simulink model "HIL_Testing_SW"  (Simulink 7.5)
settings: Solver=ode1  StartTime=0.0  StopTime=Inf  FixedStep=0.001  RelTol=1e-3
PostLoadFcn:
  | , if any(exist('dsrtsu_mdlpostloadfcn', 'file') == [2, 3, 6]), try dsrtsu_mdlpostloadfcn('Execute', bdroot); catch fprintf('Error in PostLoadFcn (dsrtsu_mdlpostloadfcn) for model "%s":\n %s\n', bdroot, lasterr); end, end,
undefined symbols (not defined in the file): CeBSER_Cnt_NumTempAxisPts, ChargeCord, ChargeCord_Control, ChargeToSOCCurr, ChrgCurrLim, CrntSens1Fine, CS_SOCSetPt, CyclerMaxChrgPwr, CyclerMaxDschrgPwr, deltaAhr, Drive_1, Drive_10, Drive_11, Drive_12, Drive_13, Drive_14, Drive_15, Drive_16, Drive_17, Drive_18, Drive_19, Drive_2, Drive_20, Drive_21, Drive_22, Drive_23, Drive_24, Drive_25, Drive_26, Drive_27, Drive_28, Drive_29, Drive_3, Drive_30, Drive_31, Drive_32, Drive_33, Drive_34, Drive_35, Drive_36, Drive_37, Drive_38, Drive_39, Drive_4, Drive_40, Drive_41, Drive_42, Drive_43, Drive_44, Drive_45, Drive_46, Drive_47, Drive_48, Drive_49, Drive_5, Drive_50, Drive_51, Drive_6, Drive_7, Drive_8 ... (+50)
libraries: simulink x129, rtican x50, rti2211sailib x5, rti2211serlib x5, rti2202miolib x3
(part 21 of 23)

== system HIL_Testing_SW/LionsHeart/FeaturePresentation/Down_to_Business/DriveProfile_ModeControl/Drive_Profile/CD/Drive_49 ==
  loop_time : Inport  OutDataType=sfix(16)  OutScaling=2^0
  Enable : EnablePort
  Lookup Table : Lookup  InputValues=Drive_49(:,1)  Table=Drive_49(:,2)  OutDataType=fixdt(1, 16)  OutScaling=2^0
  Product1 : Product  OutDataType=sfix(16)  OutScaling=2^0  RndMeth=Zero
  W_kW : Constant  Value=single(1000)  OutDataType=sfix(16)  OutScaling=2^0
  Profile_Data : Outport  OutDataType=sfix(16)  OutScaling=2^0
  wires:
  loop_time/1 -> Lookup Table/1
  W_kW/1 -> Product1/2
  Lookup Table/1 -> Product1/1
  Product1/1 -> Profile_Data/1

== system HIL_Testing_SW/LionsHeart/FeaturePresentation/Down_to_Business/DriveProfile_ModeControl/Drive_Profile/CD/Drive_5 ==
  loop_time : Inport  OutDataType=sfix(16)  OutScaling=2^0
  Enable : EnablePort
  Lookup Table : Lookup  InputValues=Drive_5(:,1)  Table=Drive_5(:,2)  OutDataType=fixdt(1, 16)  OutScaling=2^0
  Product1 : Product  OutDataType=sfix(16)  OutScaling=2^0  RndMeth=Zero
  W_kW : Constant  Value=single(1000)  OutDataType=sfix(16)  OutScaling=2^0
  Profile_Data : Outport  OutDataType=sfix(16)  OutScaling=2^0
  wires:
  loop_time/1 -> Lookup Table/1
  W_kW/1 -> Product1/2
  Lookup Table/1 -> Product1/1
  Product1/1 -> Profile_Data/1

== system HIL_Testing_SW/LionsHeart/FeaturePresentation/Down_to_Business/DriveProfile_ModeControl/Drive_Profile/CD/Drive_50 ==
  loop_time : Inport  OutDataType=sfix(16)  OutScaling=2^0
  Enable : EnablePort
  Lookup Table : Lookup  InputValues=Drive_50(:,1)  Table=Drive_50(:,2)  OutDataType=fixdt(1, 16)  OutScaling=2^0
  Product1 : Product  OutDataType=sfix(16)  OutScaling=2^0  RndMeth=Zero
  W_kW : Constant  Value=single(1000)  OutDataType=sfix(16)  OutScaling=2^0
  Profile_Data : Outport  OutDataType=sfix(16)  OutScaling=2^0
  wires:
  Product1/1 -> Profile_Data/1
  Lookup Table/1 -> Product1/1
  W_kW/1 -> Product1/2
  loop_time/1 -> Lookup Table/1

== system HIL_Testing_SW/LionsHeart/FeaturePresentation/Down_to_Business/DriveProfile_ModeControl/Drive_Profile/CD/Drive_51 ==
  loop_time : Inport  OutDataType=sfix(16)  OutScaling=2^0
  Enable : EnablePort
  Lookup Table : Lookup  InputValues=Drive_51(:,1)  Table=Drive_51(:,2)  OutDataType=fixdt(1, 16)  OutScaling=2^0
  Product1 : Product  OutDataType=sfix(16)  OutScaling=2^0  RndMeth=Zero
  W_kW : Constant  Value=single(1000)  OutDataType=sfix(16)  OutScaling=2^0
  Profile_Data : Outport  OutDataType=sfix(16)  OutScaling=2^0
  wires:
  loop_time/1 -> Lookup Table/1
  W_kW/1 -> Product1/2
  Lookup Table/1 -> Product1/1
  Product1/1 -> Profile_Data/1

== system HIL_Testing_SW/LionsHeart/FeaturePresentation/Down_to_Business/DriveProfile_ModeControl/Drive_Profile/CD/Drive_6 ==
  loop_time : Inport  OutDataType=sfix(16)  OutScaling=2^0
  Enable : EnablePort
  Lookup Table : Lookup  InputValues=Drive_6(:,1)  Table=Drive_6(:,2)  OutDataType=fixdt(1, 16)  OutScaling=2^0
  Product1 : Product  OutDataType=sfix(16)  OutScaling=2^0  RndMeth=Zero
  W_kW : Constant  Value=single(1000)  OutDataType=sfix(16)  OutScaling=2^0
  Profile_Data : Outport  OutDataType=sfix(16)  OutScaling=2^0
  wires:
  Product1/1 -> Profile_Data/1
  Lookup Table/1 -> Product1/1
  W_kW/1 -> Product1/2
  loop_time/1 -> Lookup Table/1

== system HIL_Testing_SW/LionsHeart/FeaturePresentation/Down_to_Business/DriveProfile_ModeControl/Drive_Profile/CD/Drive_7 ==
  loop_time : Inport  OutDataType=sfix(16)  OutScaling=2^0
  Enable : EnablePort
  Lookup Table : Lookup  InputValues=Drive_7(:,1)  Table=Drive_7(:,2)  OutDataType=fixdt(1, 16)  OutScaling=2^0
  Product1 : Product  OutDataType=sfix(16)  OutScaling=2^0  RndMeth=Zero
  W_kW : Constant  Value=single(1000)  OutDataType=sfix(16)  OutScaling=2^0
  Profile_Data : Outport  OutDataType=sfix(16)  OutScaling=2^0
  wires:
  Product1/1 -> Profile_Data/1
  Lookup Table/1 -> Product1/1
  W_kW/1 -> Product1/2
  loop_time/1 -> Lookup Table/1

== system HIL_Testing_SW/LionsHeart/FeaturePresentation/Down_to_Business/DriveProfile_ModeControl/Drive_Profile/CD/Drive_8 ==
  loop_time : Inport  OutDataType=sfix(16)  OutScaling=2^0
  Enable : EnablePort
  Lookup Table : Lookup  InputValues=Drive_8(:,1)  Table=Drive_8(:,2)  OutDataType=fixdt(1, 16)  OutScaling=2^0
  Product1 : Product  OutDataType=sfix(16)  OutScaling=2^0  RndMeth=Zero
  W_kW : Constant  Value=single(1000)  OutDataType=sfix(16)  OutScaling=2^0
  Profile_Data : Outport  OutDataType=sfix(16)  OutScaling=2^0
  wires:
  Product1/1 -> Profile_Data/1
  Lookup Table/1 -> Product1/1
  W_kW/1 -> Product1/2
  loop_time/1 -> Lookup Table/1

== system HIL_Testing_SW/LionsHeart/FeaturePresentation/Down_to_Business/DriveProfile_ModeControl/Drive_Profile/CD/Drive_9 ==
  loop_time : Inport  OutDataType=sfix(16)  OutScaling=2^0
  Enable : EnablePort
  Lookup Table : Lookup  InputValues=Drive_9(:,1)  Table=Drive_9(:,2)  OutDataType=fixdt(1, 16)  OutScaling=2^0
  Product1 : Product  OutDataType=sfix(16)  OutScaling=2^0  RndMeth=Zero
  W_kW : Constant  Value=single(1000)  OutDataType=sfix(16)  OutScaling=2^0
  Profile_Data : Outport  OutDataType=sfix(16)  OutScaling=2^0
  wires:
  loop_time/1 -> Lookup Table/1
  W_kW/1 -> Product1/2
  Lookup Table/1 -> Product1/1
  Product1/1 -> Profile_Data/1

== system HIL_Testing_SW/LionsHeart/FeaturePresentation/Down_to_Business/DriveProfile_ModeControl/Drive_Profile/CD/Magic ==
  note: upper
  note: Lower
  InputPower : Inport  OutDataType=fixdt(1, 16)  OutScaling=2^0
  EndTime : Inport  Port=2  OutDataType=fixdt(1, 16)  OutScaling=2^0
  LoopTime : Inport  Port=3  OutDataType=fixdt(1, 16)  OutScaling=2^0
  CD_Lo : Constant  Value=-80  OutDataType=fixdt(1, 16)  OutScaling=2^0
  CD_Up : Constant  Value=.5  OutDataType=fixdt(1, 16)  OutScaling=2^0
  CI_Lo : Constant  Value=-.5  OutDataType=fixdt(1, 16)  OutScaling=2^0
  CI_Up : Constant  Value=10  OutDataType=fixdt(1, 16)  OutScaling=2^0
  CS_Lo : Constant  Value=-5  OutDataType=fixdt(1, 16)  OutScaling=2^0
  CS_Up : Constant  Value=5  OutDataType=fixdt(1, 16)  OutScaling=2^0
  Compare To Zero : simulink/Logic and Bit Operations/Compare To Zero  SystemSampleTime=-1  relop=>=  LogicOutDataTypeMode=uint8
  Compare To Zero1 : simulink/Logic and Bit Operations/Compare To Zero  SystemSampleTime=-1  relop=>  LogicOutDataTypeMode=uint8
  Compare To Zero2 : simulink/Logic and Bit Operations/Compare To Zero  SystemSampleTime=-1  relop=>=  LogicOutDataTypeMode=uint8
  Compare To Zero3 : simulink/Logic and Bit Operations/Compare To Zero  SystemSampleTime=-1  relop=<  LogicOutDataTypeMode=uint8
  Constant{,1..2,4} (4 alike) : Constant  OutDataType=fixdt(1, 16)  OutScaling=2^0
  Constant3 : Constant  Value=.001  OutDataType=fixdt(1, 16)  OutScaling=2^0
  Data Store Read : DataStoreRead  DataStoreName=ProfileDynamicGainEnable  SampleTime=0
  Data Store Read1 : DataStoreRead  DataStoreName=ProfileChargeDesignation  SampleTime=0
  Data Store Read2 : DataStoreRead  DataStoreName=ProfileChargeDesignation  SampleTime=0
  Data Store Read3 : DataStoreRead  DataStoreName=Ahr  SampleTime=0
  Divide : Product  Inputs=*/  OutDataType=fixdt(1, 16)  OutScaling=2^-10
  Divide1 : Product  Inputs=*/  OutDataType=fixdt(1, 16)  OutScaling=2^-10
  Lookup Table1 : Lookup  InputValues=[.1 .5 .75 1 2]  Table=[-.5 0 .5 1 1]  OutDataType=fixdt(1, 16)  OutScaling=2^0
  Lookup Table2 : Lookup  InputValues=[.1 .5 .75 1 2]  Table=[-.5 0 .5 1 1]  OutDataType=fixdt(1, 16)  OutScaling=2^0
  Multiport Switch : MultiPortSwitch  zeroidx=off  OutDataType=fixdt(1, 16)  OutScaling=2^0
  Multiport Switch1 : MultiPortSwitch  zeroidx=off  OutDataType=fixdt(1, 16)  OutScaling=2^0
  Product : Product  OutDataType=fixdt(1, 16)  OutScaling=2^0  RndMeth=Zero
  Product1 : Product  OutDataType=fixdt(1, 16)  OutScaling=2^0  OutDataTypeStr=Inherit: Inherit via back propagation  RndMeth=Zero
  Relational Operator : RelationalOperator  Operator===  LogicOutDataTypeMode=boolean  LogicDataType=fixdt(0, 8)  OutDataTypeStr=boolean
  Saturation : Saturate  UpperLimit=1  LowerLimit=-1  OutDataType=fixdt(1, 16)  OutScaling=2^0
  Saturation1 : Saturate  UpperLimit=1  LowerLimit=-1  OutDataType=fixdt(1, 16)  OutScaling=2^0
  Subtract : Sum  Inputs=+-+  OutDataType=fixdt(1, 16)  OutScaling=2^-10
  Switch{,1..2,4..5} (5 alike) : Switch  Threshold=.5  OutDataType=fixdt(1, 16)  OutScaling=2^0
  Switch3 : Switch  Threshold=.5  OutDataType=fixdt(1, 16)  OutScaling=2^0  OutDataTypeStr=Inherit: Inherit via back propagation
  Unit Delay : UnitDelay  SampleTime=-1
  ProfileData : Outport  OutDataType=fixdt(1, 16)  OutScaling=2^0
  wires:
  InputPower/1 -> [InPower]
  EndTime/1 -> Relational Operator/1
  LoopTime/1 -> Relational Operator/2
  Relational Operator/1 -> Switch/2
  [Ahr] -> Switch/1
  Switch/1 -> [AhrOld], Unit Delay/1
  Unit Delay/1 -> Switch/3
  [Ahr] -> Subtract/1
  [AhrOld] -> Subtract/2
  Subtract/1 -> [AhrInternal]
  [InPower] -> Compare To Zero/1
  Compare To Zero/1 -> Switch1/2
  Constant/1 -> Switch1/1
  Constant1/1 -> Switch1/3
  [InPower] -> Product/2
  [InPower] -> Compare To Zero2/1
  Compare To Zero2/1 -> Switch2/2
  [ChargeGain] -> Switch2/1
  Switch1/1 -> Product/1
  CI_Up/1 -> Multiport Switch/2
  CS_Up/1 -> Multiport Switch/3
  CD_Up/1 -> Multiport Switch/4
  Data Store Read1/1 -> Multiport Switch/1
  Data Store Read2/1 -> Multiport Switch1/1
  CI_Lo/1 -> Multiport Switch1/2
  CS_Lo/1 -> Multiport Switch1/3
  CD_Lo/1 -> Multiport Switch1/4
  Multiport Switch/1 -> Divide/1
  Saturation/1 -> [ChargeGain]
  Multiport Switch1/1 -> Divide1/1
  Saturation1/1 -> [DisChargeGain]
  [DisChargeGain] -> Switch2/3
  Product/1 -> Switch3/1, [PowerTemp]
  [PowerTemp] -> Product1/2
  Switch2/1 -> Product1/1
  Product1/1 -> Switch3/3
  Switch3/1 -> ProfileData/1
  Constant3/1 -> Subtract/3
  Data Store Read/1 -> Switch3/2
  Data Store Read3/1 -> [Ahr]
  [AhrInternal] -> Compare To Zero1/1
  Compare To Zero1/1 -> Switch4/2
  Constant2/1 -> Switch4/3
  [AhrInternal] -> Compare To Zero3/1
  Compare To Zero3/1 -> Switch5/2
  Constant4/1 -> Switch5/3
  [AhrInternal] -> Divide/2
  Divide/1 -> Switch4/1
  Switch4/1 -> Lookup Table2/1
  Lookup Table2/1 -> Saturation/1
  [AhrInternal] -> Divide1/2
  Divide1/1 -> Switch5/1
  Switch5/1 -> Lookup Table1/1
  Lookup Table1/1 -> Saturation1/1

== stateflow chart RX/Read BAS3/PID_Reads/Chart ==
  state Zach
    en: Increment = Increment +1;
  state Initialize
    en:Increment =1;
  state Zac
    en: Increment = Increment +1;
  (default) -> Initialize
  Initialize -> Zach : after(Timer,sec)
  Zach -> Zac : after(Timer,sec)
  Zac -> Initialize : after(Timer,sec)
  data: Timer input double; Increment output double

== stateflow chart TX/Tx_Cycler/TX_ABC_ChA/Chart ==
  state Zach
    en:Trigger_one =1;
    ex:Trigger_one = 0;
  state Zachashley
    en:Trigger_two = 1;
    ex:Trigger_two = 0;
  state ashley
    en:Trigger_three = 1;
    ex:Trigger_three = 0;
    Increment = Increment +1;
  state Reset
    en:Increment =1;
  state Initialize
    en:Increment =1;
  state Zach2
  state Zachashley2
  state ashley2
  (default) -> Initialize
  Zach2 -> Zachashley : after(TickTick,tick)
  Zachashley2 -> ashley : after(TickTick,tick)
  ashley2 -> Zach : after(TickTick,tick)
  ashley -> Reset [order 1] : [Increment >254]
  Initialize -> Zach
  Reset -> Zach
  Zach -> Zach2
  Zachashley -> Zachashley2
  ashley -> ashley2 [order 2]
  data: Trigger_one output double; Trigger_two output double; Trigger_three output double; TickTick input double; Increment output double

== stateflow chart TX/Tx_Cycler/TX_ABC_ChB/Chart ==
  state Zach
    en:Trigger_one =1;
    ex:Trigger_one = 0;
  state Zachashley
    en:Trigger_two = 1;
    ex:Trigger_two = 0;
  state ashley
    en:Trigger_three = 1;
    ex:Trigger_three = 0;
    Increment = Increment +1;
  state Reset
    en:Increment =1;
  state Initialize
    en:Increment =1;
  state Zach2
  state Zachashley2
  state ashley2
  (default) -> Initialize
  Zach2 -> Zachashley : after(TickTick,tick)
  Zachashley2 -> ashley : after(TickTick,tick)
  ashley2 -> Zach : after(TickTick,tick)
  ashley -> Reset [order 1] : [Increment >254]
  Initialize -> Zach
  Reset -> Zach
  Zach -> Zach2
  Zachashley -> Zachashley2
  ashley -> ashley2 [order 2]
  data: Trigger_one output double; Trigger_two output double; Trigger_three output double; TickTick input double; Increment output double

== stateflow chart TX/Tx_Cycler/Take_Cycler_Command ==
  state Handshake
    state Handshake_Done
      en: Handshake_Complete=1;
    state Hold2
    state Ping
      en: Send_Ping=1;
      exit: Send_Ping=0;
    state Hold1
    state Greeting
      en: Send_Greeting=1;
      exit: Send_Greeting=0;
    Handshake_Done -> Handshake
    (default) -> Ping
    Hold1 -> Greeting : after(500,tick)
    Ping -> Hold1 : [(Version~=0)&&(Hardware~=0)]
    Hold2 -> Handshake_Done : after(500,tick)
    Greeting -> Hold2 : [Greeting_Sent==1]
  state Init
    en:
    Send_Ping=0;
    Send_Greeting=0;
    Send_Remote_Req_B=0;
    Send_Commands=0;
    Greeting_Sent=0;
    Remote_Req_B_Sent=0;
  state Finish
    en:
    Send_Commands=1;
  state Remote
    en:
    Channel_Change_B=Channel;
    Control_From_B=0;
    Control_To_B=1;
    Send_Remote_Req_B=1;
    exit: Send_Remote_Req_B=0;
  state Local
    en:
    Handshake_Complete = 0;
    Channel_Change_B=Channel;
    Control_From_B=1;
    Control_To_B=0;
    Send_Remote_Req_B=1;
    exit: Send_Remote_Req_B=0;
  state Wait
    en:
    Send_Ping=0;
    Send_Greeting=0;
    Send_Remote_Req_B=0;
    Send_Commands=0;
    Greeting_Sent=0;
    Remote_Req_B_Sent=0;
    Handshake_Complete = 0;
  Remote -> Handshake [order 1] : after(5000,tick)[(Remote_Req_B_Sent)&&(Side_B_Status==0)]
  Remote -> Finish [order 2] : after(100,tick)[(Remote_Req_B_Sent==1)&&(Side_B_Status==1)]
  Handshake -> Remote : [(Handshake_Complete==1)&&(Status==1)]
  (default) -> Init
  Init -> Handshake : [Perform_Handshake]
  Finish -> Local : [Reset_to_Local == 1]
  Local -> Wait : [Side_B_Status==0]
  Wait -> Handshake : [Perform_Handshake]
  data: Version input double; Hardware input double; Status input double; Send_Ping output double; Send_Greeting output double; Greeting_Sent data_store_memory double; Send_Remote_Req_B output double; Side_B_Status input double; Perform_Handshake input boolean; Handshake_Complete data_store_memory double; Remote_Req_B_Sent data_store_memory double; Channel_Change_B output double; Control_From_B output double; Control_To_B output double; Send_Commands output double =0; Reset_to_Local input boolean; Channel input double

== stateflow chart TX/Chiller/ChillerCmndTxDecision/ChillerStateFlow ==
  state EvaluateChillerOnOff
  state ManualSelect
    en:
    WaitRx = 1;
    ChillerTx = ManualChillerSP_Cmnd;
    ChillerTxNumBytes = 8;
    ChillerRxNumBytes = 2;
    exit:
    ChillerTxNumBytes = 0;
  state ReadChillerSP2
    en:
    exit:
    ReadChillerSP_Action = 0;
  state TurnChillerOff
    en:
    WaitRx = 1;
    ChillerTx = TurnChiller_Off;
    ChillerTxNumBytes = 4;
    ChillerRxNumBytes = 2;
  state GoBack
  state ReadChillerTemp2
    en:
    exit:
    ReadChillerTemp_Action = 0;
  state ManualSelect1
    en:
    exit:
    ChillerTxNumBytes = 0;
    WaitRx = 0;
  state ReadChillerStatus1
    en:
    WaitRx = 0;
    ReadChillerStatus_Action = 1;
    ChillerTx = ReadChillerStatus;
    ChillerTxNumBytes = 3;
    ChillerRxNumBytes = 2;
  state ReadChillerSP1
    en:
    ChillerTx = ReadChillerSP;
    ChillerTxNumBytes = 3;
    ChillerRxNumBytes = 7;
    ReadChillerSP_Action = 1;
    exit:
    ChillerTxNumBytes = 0;
  state ReadChillerTemp1
    en:
    ReadChillerTemp_Action = 1;
    ChillerTx = ReadChillerTemp;
    ChillerTxNumBytes = 3;
    ChillerRxNumBytes = 7;
    exit:
    ChillerTxNumBytes = 0;
  state EvaluateBatTemp3
    en:
    WaitRx = 1;
    ChillerTx = TurnChiller_On;
    ChillerTxNumBytes = 4;
    ChillerRxNumBytes = 2;
    exit:
    ChillerTxNumBytes = 0;
  state EvaluateBatTemp4
    en:
    WaitRx = 0;
    ChillerTxNumBytes = 0;
    ChillerRxNumBytes = 0;
    ChillerPowerStatus = 0;
  state ReadChillerStatus
    en:
    exit:
    ReadChillerStatus_Action = 0;
    ChillerPowerStatus = 1;
  state FollowProfileTemp
    en:
    WaitRx = 1;
    ChillerTx =  BatTempSwitchSlct;
    ChillerTxNumBytes = 8;
    ChillerRxNumBytes = 2;
    exit:
    ChillerTxNumBytes = 0;
  (default) -> EvaluateBatTemp4
  EvaluateBatTemp4 -> EvaluateBatTemp3 [order 1] : [(ChillerOnOff == 1 && (BatTemp > 33 || BatTemp < 0) && ChillerOpMode ==1)]
  EvaluateChillerOnOff -> FollowProfileTemp [order 2] : [(ChillerOpMode == 1 && (BatTemp > 33 || BatTemp < 0))]
  EvaluateChillerOnOff -> ManualSelect [order 4] : [ChillerOpMode == 3&&ManualChillerPower ==1]
  EvaluateChillerOnOff -> ManualSelect [order 3] : [(ChillerOpMode == 2&&ManualChillerPower ==1)]
  ManualSelect1 -> ReadChillerSP1
  EvaluateChillerOnOff -> TurnChillerOff [order 1] : [(ChillerOnOff == 0)&&(ChillerOpMode == 1)]
  ReadChillerTemp1 -> ReadChillerTemp2
  ReadChillerSP2 -> ReadChillerTemp1
  ManualSelect -> ManualSelect1 : [PositiveResponse == 1]
  EvaluateBatTemp3 -> ReadChillerStatus1 : [PositiveResponse == 1]
  TurnChillerOff -> EvaluateBatTemp4 : [PositiveResponse == 1]
  ReadChillerSP1 -> ReadChillerSP2
  (junction 123) -> EvaluateChillerOnOff
  GoBack -> EvaluateChillerOnOff
  EvaluateChillerOnOff -> TurnChillerOff [order 6] : [(ChillerOpMode == 1 && BatTemp >= 0 && BatTemp < 33)]
  FollowProfileTemp -> ManualSelect1 : [PositiveResponse == 1]
  ReadChillerStatus1 -> ReadChillerStatus : [ChillerOn == 1]
  ReadChillerStatus -> (junction 122)
  (junction 122) -> (junction 123)
  EvaluateBatTemp4 -> EvaluateBatTemp3 [order 2] : [ChillerOpMode == 3]
  ReadChillerTemp2 -> GoBack
  EvaluateChillerOnOff -> TurnChillerOff [order 5] : [ManualChillerPower == 0]
  EvaluateBatTemp4 -> EvaluateBatTemp3 [order 3] : [ManualChillerPower == 1]
  data: BatTempSwitchSlct input uint8 size=8; ManualChillerSP_Cmnd input uint8 size=8; ChillerTx output uint8 size=8; ChillerTxNumBytes output uint32; ChillerRxNumBytes output uint32; ReadChillerSP_Action output boolean; ChillerOnOff input boolean; ChillerOpMode input uint8; TurnChiller_On input uint8 size=8; TurnChiller_Off input uint8 size=8; ReadChillerSP input uint8 size=8; ReadChillerTemp input uint8 size=8; ReadChillerTemp_Action output boolean; PositiveResponse input boolean size=1; ReadChillerStatus input uint8 size=8; ChillerOn input boolean; ReadChillerStatus_Action output boolean; ManualChillerPower input boolean; ChillerPowerStatus output boolean; WaitRx output boolean; BatTemp input single

== stateflow chart LionsHeart/FeaturePresentation/Down_to_Business/DriveProfile_ModeControl/Capacity Test/Capacity_Test ==
  state ChargeTerminate
    entry:
    Mode_Cntrl_cap = 1;
    Step=5;
    WaitTime=0;
    RateInternal = RateInternal*RateFactor;
    ChrgCurrLim_Tmp=RateInternal;
    Control_Value_cap = RateInternal;
    du:
    WaitTime=WaitTime+sim_step_time;
    ChrgCurrLim_Tmp=RateInternal;
    Control_Value_cap = RateInternal;
    Cappy = 7;
  state DischargeTerminate
    entry:
    WaitTime = 0;
    Mode_Cntrl_cap = 1;
    Step=2;
    RateInternal = RateInternal*RateFactor;
    DischrgCurrLim_Tmp = RateInternal;
    Control_Value_cap = RateInternal
    du:
    DischrgCurrLim_Tmp = RateInternal;
    Control_Value_cap = RateInternal;
    WaitTime=WaitTime+sim_step_time;
    Cappy = 3;
  state Taper
    entry:
    WaitTime = 0;
    du:
    WaitTime = WaitTime + sim_step_time;
    Cappy = 4;
  state Rest2
    entry:
    ResetSOCFlg = 1;
    Mode_Cntrl_cap = 3;
    WaitTime =0;
    Step=6;
    during:
    ResetSOCFlg = 0;
    WaitTime = WaitTime + sim_step_time;
    Cappy = 9;
    exit:
    cycle = cycle+1;
  state end_test
    entry:
    Step=99;
    Mode_Cntrl_cap = 3;
    DischrgCurrLim_Tmp=DischrgCurrLim;
    ChrgCurrLim_Tmp=ChrgCurrLim;
  state Taper_Charge
    entry:
    WaitTime = 0;
    du:
    WaitTime = WaitTime + sim_step_time;
    Cappy = 8;
  state Charge
    entry:
    Mode_Cntrl_cap = 1;
    Step=4;
    WaitTime=0;
    du:
    RateInternal = CRate;
    WaitTime=WaitTime+sim_step_time;
    ChrgCurrLim_Tmp=CRate;
    Control_Value_cap = CRate;
    Cappy = 6;
  state start_test
    entry:
    Step=0;
    cycle = 0;
    Mode_Cntrl_cap = 3;
    WaitTime = 0;
    DischrgCurrLim_Tmp=DischrgCurrLim;
    ChrgCurrLim_Tmp=ChrgCurrLim;
    ContactorOverride =1;
    du:
    WaitTime=WaitTime+sim_step_time;
    Cappy = 1;
  state Rest
    entry:
    ResetSOCFlg = 1;
    Mode_Cntrl_cap = 3;
    WaitTime =0;
    Step=3;
    during:
    WaitTime = WaitTime + sim_step_time;
    Cappy = 5;
    ResetSOCFlg = 0;
  state discharge
    entry:
    WaitTime = 0;
    Mode_Cntrl_cap = 1;
    Step=1;
    DischrgCurrLim_Tmp = -1*CRate;
    Control_Value_cap = -1*CRate;
    du:
    RateInternal = -1*CRate;
    DischrgCurrLim_Tmp = -1*CRate;
    Control_Value_cap = -1*CRate;
    WaitTime=WaitTime+sim_step_time;
    Cappy = 2;
  (default) -> start_test
  ChargeTerminate -> Rest2 [order 1] : [((Current_Cntrl<=CurrentTerm) && (WaitTime >=2)) || (CyclerVoltage > Vlid)]
  Taper_Charge -> ChargeTerminate [order 2] : [((Voltage_Cntrl>=Vlid) || ((PackVolt_MaxCell>=Vlid_cell) && (MaxCell_Enbl == 1))) && WaitTime > .5]
  ChargeTerminate -> Taper_Charge [order 2]
  DischargeTerminate -> Rest [order 1] : [((Current_Cntrl >=-1*CurrentTerm) && (WaitTime >= .5)) || (CyclerVoltage< Vfloor)]
  DischargeTerminate -> Taper [order 2]
  Taper -> DischargeTerminate [order 2] : [((Voltage_Cntrl<=Vfloor) || ((PackVolt_MinCell <=Vfloor_cell) && MinCell_Enbl == 1)) && (WaitTime > .5)]
  Rest2 -> discharge [order 2] : [ (WaitTime >= RestTime) && (cycle<NumberCycles)]
  discharge -> Rest [order 2] : [((Voltage_Cntrl<= Vfloor) || ((PackVolt_MinCell <=Vfloor_cell) && (MinCell_Enbl == 1))) && (Vfloor != OCV_Zero)]
  Rest -> Charge : [ WaitTime >= RestTime]
  discharge -> DischargeTerminate [order 1] : [((Voltage_Cntrl<=Vfloor) || ((PackVolt_MinCell <=Vfloor_cell) && (MinCell_Enbl == 1))) && (Vfloor == OCV_Zero)]
  start_test -> discharge : [ (cycle < NumberCycles) && (WaitTime>=30)]
  Charge -> ChargeTerminate : [(Voltage_Cntrl>=Vlid) || ((PackVolt_MaxCell>=Vlid_cell) && (MaxCell_Enbl == 1))]
  Rest2 -> end_test [order 1] : [(WaitTime >= RestTime) && (cycle>=NumberCycles)]
  Taper -> Rest [order 1] : [Current_Cntrl >=-1*CurrentTerm]
  Taper_Charge -> Rest2 [order 1] : [Current_Cntrl<=CurrentTerm]
  data: Control_Value_cap output double; Vfloor input single; WaitTime output double; Mode_Cntrl_cap output single; Vlid input single; CurrentTerm input single; Voltage_Cntrl input single; Current_Cntrl input single; NumberCycles input single; sim_step_time input single; cycle output single; RestTime input single; ChrgCurrLim input single; DischrgCurrLim input single; DischrgCurrLim_Tmp output single; ChrgCurrLim_Tmp output single; Step output single; PackVolt_MinCell input double; PackVolt_MaxCell input double; RateFactor input single; Vfloor_cell input double; Vlid_cell input double; MaxCell_Enbl input double; MinCell_Enbl input double; CyclerVoltage input double; RateInternal local double; OCV_Zero input double; CRate input double; ContactorOverride output double; Cappy output int32; ResetSOCFlg output boolean

== stateflow chart LionsHeart/FeaturePresentation/Down_to_Business/DriveProfile_ModeControl/Charging_Mode/Charging Logic1 ==
  state WaitBlock2
    Step =7;
    WaitTime = 0;
    du:
    WaitTime = WaitTime + sim_step_time;
  state CheckDirectionVoltage
    entry:
    Mode_Cntrl_cap=3;
  state Pack_Sens_Termination3
    entry:
    Mode_Cntrl_cap = 3;
    WaitTime= 0;
    Step=0;
    du:
    WaitTime=WaitTime+sim_step_time;
    DisChrgCurr_Limit = DisChrgCurrLimit_Cal;
    ChargeLimit_Temp = ChargeLimitCal;
  state Pack_Sens_DschrgTerminate
    entry:
    Mode_Cntrl_cap = 1;
    Step=6;
    RateDschrg= RateDschrg*RateFactor;
    Control_Value_cap = RateDschrg;
    du:
    Control_Value_cap = RateDschrg;
  state Pack_Sens_Discharge
    entry:
    RateChrgInternal = RateChrg;
    RateDschrg = RateChrg*-1;
    DisChrgCurr_Limit = RateDschrg;
    ChargeLimit_Temp = RateChrgInternal;
    Mode_Cntrl_cap = 1;
    Step=2;
    du:
    Control_Value_cap = RateDschrg;
  state Decision_Block
    Mode_Cntrl_cap = 3;
  state Pack_Sens_Termination2
    entry:
    Step=99;
    Mode_Cntrl_cap = 3;
    DisChrgCurr_Limit = DisChrgCurrLimit_Cal;
    ChargeLimit_Temp = ChargeLimitCal;
    du:
    Mode_Cntrl_cap = 3;
    DisChrgCurr_Limit = DisChrgCurrLimit_Cal;
    ChargeLimit_Temp = ChargeLimitCal;
  state Pack_Sens_Termination
    entry:
    Mode_Cntrl_cap = 1;
    Step=6;
    RateChrgInternal = RateChrgInternal *RateFactor;
    Control_Value_cap = RateChrgInternal;
    du:
    Control_Value_cap = RateChrgInternal;
  state Pack_Sens_Termination1
    entry:
    RateChrgInternal = RateChrg;
    DisChrgCurr_Limit = RateChrgInternal*-1;
    ChargeLimit_Temp = RateChrgInternal;
    Mode_Cntrl_cap = 1;
    Step=2;
    du:
    RateChrgInternal = RateChrg;
    Control_Value_cap = RateChrgInternal;
  state WaitBlock1
    Step =7;
    WaitTime = 0;
    du:
    WaitTime = WaitTime + sim_step_time;
  state CheckDirectionSOC
    entry:
    Mode_Cntrl_cap=3;
  state Termination_SOC
    entry:
    Step=99;
    Mode_Cntrl_cap = 3;
    DisChrgCurr_Limit = DisChrgCurrLimit_Cal;
    ChargeLimit_Temp = ChargeLimitCal;
    du:
    Mode_Cntrl_cap = 3;
    DisChrgCurr_Limit = DisChrgCurrLimit_Cal;
    ChargeLimit_Temp = ChargeLimitCal;
  state TaperToCurrentTerm_SOC
    entry:
    Mode_Cntrl_cap = 1;
    Step=6;
    RateChrgInternal = RateChrgInternal *RateFactor;
    Control_Value_cap = RateChrgInternal;
    du:
    Control_Value_cap = RateChrgInternal;
  state ChargeToSOC
    entry:
    RateChrgInternal = RateChrg;
    DisChrgCurr_Limit = RateChrgInternal*-1;
    ChargeLimit_Temp = RateChrgInternal;
    Mode_Cntrl_cap = 1;
    Step=2;
    du:
    RateChrgInternal = RateChrg;
    Control_Value_cap = RateChrgInternal;
  state WaitBlock3
    Step =7;
    WaitTime = 0;
    du:
    WaitTime = WaitTime + sim_step_time;
  state WaitBlock4
    Step =7;
    WaitTime = 0;
    du:
    WaitTime = WaitTime + sim_step_time;
  state Pack_Sens_DschrgTerminate1
    entry:
    Mode_Cntrl_cap = 1;
    Step=6;
    RateDschrg= RateDschrg*RateFactor;
    Control_Value_cap = RateDschrg;
    du:
    Control_Value_cap = RateDschrg;
  state DischargeToSOC
    entry:
    RateChrgInternal = RateChrg;
    RateDschrg = RateChrg*-1;
    DisChrgCurr_Limit = RateDschrg;
    ChargeLimit_Temp = RateChrgInternal;
    Mode_Cntrl_cap = 1;
    Step=2;
    du:
    Control_Value_cap = RateDschrg;
  (default) -> Decision_Block
  Pack_Sens_DschrgTerminate -> Pack_Sens_Termination2 [order 1] : [(Current_Cntrl>=-1*CurrentTerm) || (CyclerVoltage<VFloor)]
  Pack_Sens_Termination3 -> CheckDirectionVoltage [order 2] : [(WaitTime >= WaitTime1) && ((ChargeSelect == 0) || (ChargeSelect==1))]
  Pack_Sens_DschrgTerminate -> WaitBlock2 [order 2]
  CheckDirectionVoltage -> Pack_Sens_Termination1 [order 1] : [Voltage_Cntrl<=VoltageSetPoint]
  WaitBlock2 -> Pack_Sens_DschrgTerminate [order 2] : [((PackVoltage_MinCell<=VoltageSetPoint) && (MinCell_Enbl == 1)) || (CyclerVoltage <= VoltageSetPoint) || (Voltage_Cntrl<=VoltageSetPoint)&& (WaitTime > .5)]
  Pack_Sens_Discharge -> Pack_Sens_DschrgTerminate : [((PackVoltage_MinCell<=VoltageSetPoint) && (MinCell_Enbl == 1)) || (CyclerVoltage <= VoltageSetPoint) || (Voltage_Cntrl<=VoltageSetPoint)]
  CheckDirectionVoltage -> Pack_Sens_Discharge [order 2] : [Voltage_Cntrl>VoltageSetPoint]
  WaitBlock1 -> Pack_Sens_Termination [order 2] : [(((PackVoltage_MaxCell>=VoltageSetPt_Max) && (MaxCell_Enbl == 1)) || (CyclerVoltage>=(VoltageSetPoint+CyclerOffset)) || (Voltage_Cntrl >= VoltageSetPoint)) && (WaitTime > .5)]
  Pack_Sens_Termination -> Pack_Sens_Termination2 [order 1] : [(Current_Cntrl<CurrentTerm) || (CyclerVoltage>(VoltageLid+CyclerOffset))]
  Pack_Sens_Termination1 -> Pack_Sens_Termination : [((PackVoltage_MaxCell >= VoltageSetPt_Max) && (MaxCell_Enbl ==1)) || (CyclerVoltage >= VoltageSetPoint) || (Voltage_Cntrl >=VoltageSetPoint)]
  Pack_Sens_Termination -> WaitBlock1 [order 2]
  Decision_Block -> Pack_Sens_Termination3
  WaitBlock1 -> Pack_Sens_Termination2 [order 1] : [Current_Cntrl<CurrentTerm]
  WaitBlock2 -> Pack_Sens_Termination2 [order 1] : [Current_Cntrl>=-1*CurrentTerm]
  Pack_Sens_Termination3 -> CheckDirectionSOC [order 1] : [(WaitTime >= WaitTime1) && (ChargeSelect == 2)]
  CheckDirectionSOC -> ChargeToSOC [order 1] : [SOC<=SOCTarget]
  WaitBlock3 -> TaperToCurrentTerm_SOC [order 2] : [((SOC>=SOCTarget) && (WaitTime > .5))]
  TaperToCurrentTerm_SOC -> Termination_SOC [order 1] : [(Current_Cntrl<CurrentTerm) || (CyclerVoltage>VoltageLid)]
  ChargeToSOC -> TaperToCurrentTerm_SOC : [SOC>=SOCTarget]
  TaperToCurrentTerm_SOC -> WaitBlock3 [order 2]
  WaitBlock3 -> Termination_SOC [order 1] : [Current_Cntrl<CurrentTerm]
  CheckDirectionSOC -> Termination_SOC [order 2] : [SOC >! 0]
  Pack_Sens_DschrgTerminate1 -> Termination_SOC [order 1] : [(Current_Cntrl>=-1*CurrentTerm) || (CyclerVoltage<VFloor)]
  Pack_Sens_DschrgTerminate1 -> WaitBlock4 [order 2]
  WaitBlock4 -> Pack_Sens_DschrgTerminate1 [order 2] : [((SOC<=SOCTarget) && (WaitTime > .5))]
  DischargeToSOC -> Pack_Sens_DschrgTerminate1 : [SOC<=SOCTarget]
  CheckDirectionSOC -> DischargeToSOC [order 3] : [SOC>SOCTarget]
  WaitBlock4 -> Termination_SOC [order 1] : [Current_Cntrl>=-1*CurrentTerm]
  data: Control_Value_cap output double; WaitTime output double; RateChrg input single; Mode_Cntrl_cap output single; VoltageSetPoint input single; CurrentTerm input single; Current_Cntrl input single; sim_step_time input single; WaitTime1 input single; ChargeSelect input single; SOC input double; VoltageLid input single; ChargeLimitCal input single; ChargeLimit_Temp output single; DisChrgCurr_Limit output single; DisChrgCurrLimit_Cal input single; Step output double; RateChrgInternal local double; CyclerVoltage input single; SOCTarget input double; RateFactor input single; VFloor input single; PackVoltage_MaxCell input double; PackVoltage_MinCell input double; RateDschrg local double; VoltageSetPt_Max input double; Voltage_Cntrl input double; MaxCell_Enbl input double; MinCell_Enbl input double; CyclerOffset input double

== stateflow chart LionsHeart/FeaturePresentation/Down_to_Business/DriveProfile_ModeControl/Drive_Profile/CD/Power_Cycle_Timer ==
  state start_dvr
    entry:
    loop_counter = 0;
    loop_time = 0;
  state run_cycle
    entry:loop_time = StartTime;
    during:
    loop_time = loop_time + sim_time_step;
    exit:
    loop_time = 0;
  state End_Test
    entry:
    loop_time = 0;
  state run_cycle1
    during:
    loop_time = loop_time + sim_time_step;
    exit:
    loop_time = 0;
  (default) -> start_dvr
  run_cycle -> start_dvr [order 1] : [ cycle_enable == 0]
  run_cycle -> End_Test [order 2] : [ loop_time >= cycle_duration ]
  start_dvr -> run_cycle [order 1] : [ (cycle_enable  == 1) && (StartTime~=0) ]
  End_Test -> start_dvr : [ cycle_enable == 0]
  start_dvr -> run_cycle1 [order 2] : [(cycle_enable==1) && (StartTime==0)]
  run_cycle1 -> start_dvr [order 1] : [cycle_enable ==0]
  run_cycle1 -> End_Test [order 2] : [loop_time>=cycle_duration]
  data: loop_counter output double; cycle_enable input boolean; sim_time_step input double; cycle_duration input double; loop_time output double; StartTime input double

== stateflow chart LionsHeart/FeaturePresentation/Down_to_Business/DriveProfile_ModeControl/HPPC Test/HPPC_Test ==
  state start_test
    entry:
    cycle = 0;
    ChrgCurrLim_Tmp=ChrgCurrLim;
  state Rest
    entry:
    RestTime =0;
    Mode_Cntrl = 3;
    Step=2;
    during:
    RestTime = RestTime + sim_step_time;
  state First_Discharge
    entry:
    EndTime = 0;
    during:
    Mode_Cntrl = 1;
    Step=3;
    Control_Value = RateDischrg;
    EndTime = EndTime + sim_step_time;
  state Discharge_Pulse
    entry:
    PulseTime=0;
    Step=4;
    du:
    Mode_Cntrl = 1;
    Control_Value = DischrgPulseCurr;
    PulseTime = PulseTime + sim_step_time;
  state Charge_Pulse
    entry:
    PulseTime =0;
    Step=4;
    during:
    PulseTime = PulseTime + sim_step_time;
    Mode_Cntrl = 1;
    Control_Value = ChrgPulseCurr;
  state Rest_Btwn_Pulse
    entry:
    RestBtwnTime =0;
    Mode_Cntrl = 3;
    Step=2;
    during:
    RestBtwnTime = RestBtwnTime + sim_step_time;
  state end_test
    entry:
    Mode_Cntrl = 3;
    Step=7;
  state Rest_Before
    entry:
    RestBefore =0;
    Mode_Cntrl = 3;
    Step=2;
    during:
    RestBefore = RestBefore + sim_step_time;
  state Discharge%
    entry:
    EndTime2 = 0;
    Step=3;
    during:
    Mode_Cntrl = 1;
    Control_Value = RateDischrg;
    EndTime2 = EndTime2 + sim_step_time;
  state LongRest
    entry:
    LongRest =0;
    Mode_Cntrl = 3;
    Step=6;
    during:
    LongRest = LongRest + sim_step_time;
    ex:
    cycle=1;
  state DischargeResidual
    entry:
    Mode_Cntrl = 1;
    Step=5;
    during:
    Control_Value = RateDischrg;
  state Charge
    entry:
    Mode_Cntrl = 1;
    Step=1
    WaitTime=0;
    du:
    ChrgCurrLim_Tmp = RateChrg;
    Control_Value = VoltageTerm;
    WaitTime= WaitTime+ sim_step_time;
  state LongRestConditon
    entry:
    LongRest =0;
    Mode_Cntrl = 3;
    Step=21;
    during:
    LongRest = LongRest + sim_step_time;
  state RestShort
    entry:
    Mode_Cntrl = 3;
    RestShort =0;
    Step=1;
    during:
    RestShort = RestShort + sim_step_time;
  (default) -> start_test
  Rest -> Discharge_Pulse : [ RestTime >= RestTimeSet]
  First_Discharge -> Rest : [EndTime>=DischrgTime]
  LongRestConditon -> First_Discharge : [LongRest>=LongRestSet]
  Discharge_Pulse -> Rest_Btwn_Pulse : [PulseTime >= PulseTimeSet]
  Charge_Pulse -> Rest_Before : [PulseTime>=PulseTimeSet]
  Rest_Btwn_Pulse -> Charge_Pulse : [RestBtwnTime >= BtwnTimeSet]
  Charge -> end_test [order 1] : [(cycle>=1)&& (Current<=CurrentTerm)]
  Rest_Before -> Discharge% : [RestBefore>=RestBeforeSet]
  Discharge% -> Rest [order 1] : [EndTime2>=DischrgTime2]
  DischargeResidual -> LongRest : [Voltage<=VoltageFloor]
  Discharge% -> DischargeResidual [order 2] : [Voltage<=(VoltageFloor+0.5)]
  LongRest -> RestShort : [LongRest>=LongRestSet]
  start_test -> RestShort
  RestShort -> Charge : [RestShort>=RestShortSet]
  Charge -> LongRestConditon [order 2] : [(Current<=CurrentTerm) && (cycle<1) && (WaitTime>=30)]
  data: Control_Value output double; RestShort local single; RateDischrg input single; LongRest local double; RateChrg input single; Mode_Cntrl output single; VoltageTerm input single; CurrentTerm input single; Voltage input single; Current input single; RestShortSet input single; sim_step_time input single; cycle local single; LongRestSet input single; RestTime local single; RestTimeSet input single; DischrgPulseCurr input single; PulseTime local single; PulseTimeSet input single; RestBtwnTime local single; BtwnTimeSet input single; ChrgPulseCurr input single; RestBefore local single; RestBeforeSet input single; EndTime local single; EndTime2 local single; DischrgTime input single; DischrgTime2 input single; VoltageFloor input single; Step output single; WaitTime local single; ChrgCurrLim input single; ChrgCurrLim_Tmp output single

== stateflow chart LionsHeart/FeaturePresentation/Down_to_Business/DriveProfile_ModeControl/Idle/Idle ==
  state DirectionDecision
    entry:
    Step =0;
  state ConstPower
    entry:
    Step =1;
    Mode_Cntrl = 2;
    Control_Value=PowerRequest*1000;
    Time = 0;
    du:
    Time = Time + sim_step_time
  state EndTime
    entry:
    Step =99
    Mode_Cntrl=3;
  state ConstCurrent
    entry:
    Step =1;
    Mode_Cntrl = 1;
    Control_Value=CurrentRequest;
    Time = 0;
    du:
    Time = Time + sim_step_time
  (default) -> DirectionDecision
  DirectionDecision -> ConstPower [order 2] : [Idle_Type==1]
  ConstPower -> EndTime : [Time >=TimeRequest]
  ConstCurrent -> EndTime : [Time >=TimeRequest]
  DirectionDecision -> ConstCurrent [order 1] : [Idle_Type==2]
  data: Control_Value output single; Mode_Cntrl output single; PowerRequest input single; CurrentRequest input single; TimeRequest input double; sim_step_time input single; Step output double; Time local double; Idle_Type input double

== stateflow chart LionsHeart/FeaturePresentation/Down_to_Business/DriveProfile_ModeControl/Increment/IncrementRate ==
  state WaitForMe
    entry:
    Wait=0;
    Mode_Cntrl =3;
    Step =3;
    du:
    Wait=Wait+sim_step_time;
  state DischrgPulse
    entry:
    Step =1;
    Mode_Cntrl = 1;
    Control_Value=Pulse;
    DschrgLimit=Pulse;
    PulseTime = 0;
    du:
    PulseTime = PulseTime + sim_step_time;
    Control_Value=Pulse;
    DschrgLimit=Pulse;
  state EndTime
    entry:
    Wait=0;
    Mode_Cntrl =3;
    Step =99;
    du:
    Wait=Wait+sim_step_time;
    exit:
    Step=2;
    DschrgLimit=DschrgCal;
  state Start
    entry:
    Step =0;
    DschrgLimit=DschrgCal;
    Mode_Cntrl=3;
  state IncrementDschrg
    entry:
    Step =4;
    Mode_Cntrl = 1;
    DschrgLimit=Increment;
    Control_Value=Increment;
    AhrOld = Ahr;
    Wait=0;
    du:
    Delta = abs(Ahr)-abs(AhrOld);
    Control_Value=Increment;
    DschrgLimit=Increment;
    Wait=Wait+sim_step_time;
  state WaitForMe1
    entry:
    Wait=0;
    Mode_Cntrl =3;
    Step =3;
    du:
    Wait=Wait+sim_step_time;
  (default) -> Start
  EndTime -> Start : [Step==99]
  DischrgPulse -> WaitForMe [order 2] : [PulseTime >=PTime]
  WaitForMe -> IncrementDschrg : [(Wait>=40)]
  Start -> DischrgPulse : after(10,sec)
  IncrementDschrg -> WaitForMe1 [order 2] : [(Delta>=deltaAhr) && (Wait>5)]
  WaitForMe1 -> DischrgPulse : [Wait>=WaitTime]
  DischrgPulse -> EndTime [order 1] : [(PackVolt_MinCell <=VfloorCell) || (Voltage <=Vfloor)]
  IncrementDschrg -> EndTime [order 1] : [(PackVolt_MinCell <= VfloorCell) || (Voltage <= Vfloor)]
  data: Control_Value output double; Mode_Cntrl output single; sim_step_time input single; Step output single; PulseTime local double; PTime input double; Wait local double; Voltage input double; PackVolt_MinCell input double; Pulse input double; Increment input double; deltaAhr input double; WaitTime input double; Ahr input double; Vfloor input double; VfloorCell input double; AhrOld local double; Delta local double; DschrgLimit output double; DschrgCal input double

== stateflow chart LionsHeart/Input Processing/Voltage Processing/ChargeTermVoltage/LookupChrgVoltageSetPoint_BSE/Stateflow Chart1 ==
  (default) -> (junction 459) : {LeBSER_i_i = 0;}
  (junction 453) -> (junction 452) [order 1] : [ VeBSER_T_HV_BatTemp < KnBSEM_T_TempAxis[LeBSER_i_i + 1] ]
  (junction 451) -> (junction 453) [order 1] : [LeBSER_i_i < CeBSER_Cnt_NumTempAxisPts]
  (junction 454) -> (junction 451) : {LeBSER_i_i++;}
  (junction 455) -> (junction 457) [order 1] : [VeBSER_T_HV_BatTemp >= KnBSEM_T_TempAxis[CeBSER_Cnt_NumTempAxisPts-1]]
  (junction 453) -> (junction 454) [order 2]
  (junction 452) -> (junction 458) : {LeBSER_i_Indx = LeBSER_i_i+1;
      | LeBSER_r_ScaleFctr = (VeBSER_T_HV_BatTemp - KnBSEM_T_TempAxis[ LeBSER_i_i ]) /(KnBSEM_T_TempAxis[ LeBSER_i_i ] - KnBSEM_T_TempAxis[ LeBSER_i_i + 1]);
      | LeBSER_i_i = CeBSER_Cnt_NumTempAxisPts;}
  (junction 451) -> (junction 456) [order 2]
  (junction 463) -> (junction 451)
  (junction 458) -> (junction 454)
  (junction 462) -> (junction 455)
  (junction 459) -> (junction 460) [order 1] : [VeBSER_T_HV_BatTemp<= KnBSEM_T_TempAxis[0]]
  (junction 460) -> (junction 461) : {LeBSER_i_Indx = 1;
      | LeBSER_r_ScaleFctr = 0.0;
      | LeBSER_i_i = CeBSER_Cnt_NumTempAxisPts;}
  (junction 459) -> (junction 462) [order 2]
  (junction 461) -> (junction 462)
  (junction 464) -> (junction 463)
  (junction 455) -> (junction 463) [order 2]
  (junction 457) -> (junction 464) : {LeBSER_i_Indx = CeBSER_Cnt_NumTempAxisPts-1;
      | LeBSER_r_ScaleFctr = -1.0;
      | LeBSER_i_i = CeBSER_Cnt_NumTempAxisPts;}
  data: LeBSER_i_i local uint32; VeBSER_T_HV_BatTemp input single; KnBSEM_T_TempAxis input single size=9; LeBSER_i_Indx output uint32; LeBSER_r_ScaleFctr output single; CeBSER_Cnt_NumTempAxisPts input uint8

== stateflow chart LionsHeart/FeaturePresentation/Down_to_Business/DriveProfile_ModeControl/OCV Test/OCV_Test ==
  state start_test
    entry:
    ResetRun=0;
    Step=0;
    Mode_Cntrl_cap = 3;
    WaitTime = 0;
    DischrgCurrLim_Tmp=DischrgCurrLim;
    ChrgCurrLim_Tmp=ChrgCurrLim;
    du:
    WaitTime=WaitTime+sim_step_time;
    ResetSOC=1;
    ex:
    ResetSOC=0;
  state RestBefore
    entry:
    ResetRun=1;
    Mode_Cntrl_cap = 3;
    WaitTime =0;
    Step=3;
    during:
    WaitTime = WaitTime + sim_step_time;
    exit: ResetRun=0;
  state discharge
    entry:
    WaitTime = 0;
    Mode_Cntrl_cap = 0;
    Step=1;
    DischrgCurrLim_Tmp = RateDischrg;
    Control_Value_cap = Vfloor;
    du:
    DischrgCurrLim_Tmp = RateDischrg;
    Control_Value_cap = Vfloor;
    WaitTime=WaitTime+sim_step_time;
    exit:DischrgCurrLim_Tmp=DischrgCurrLim;
  state Charge
    entry:
    Mode_Cntrl_cap = 0;
    Step=2;
    WaitTime=0;
    du:
    WaitTime=WaitTime+sim_step_time;
    ChrgCurrLim_Tmp=RateChrg;
    Control_Value_cap = Vlid;
    exit:ChrgCurrLim_Tmp=ChrgCurrLim;
  state end_test
    entry:
    Step=99;
    Mode_Cntrl_cap = 3;
    DischrgCurrLim_Tmp=DischrgCurrLim;
    ChrgCurrLim_Tmp=ChrgCurrLim;
  state DischargeIncrement
    entry:
    AhrOld=Ahr;
    WaitTime = 0;
    Mode_Cntrl_cap = 1;
    Step=5;
    Control_Value_cap = RateOCVDischrg;
    du:
    Control_Value_cap = RateOCVDischrg;
    Delta=abs(Ahr)-abs(AhrOld);
    WaitTime=WaitTime+sim_step_time;
  state RestBetweenResetRun
    entry:
    Mode_Cntrl_cap = 3;
    WaitTime =0;
    Step=6;
    ResetRun=1;
    during:
    WaitTime = WaitTime + sim_step_time;
    exit:ResetRun=0;
  state ResetSOC
    entry:
    Mode_Cntrl_cap = 3;
    WaitTime =0;
    Step=4;
    ResetSOC=1;
    during:
    WaitTime = WaitTime + sim_step_time;
    exit: ResetSOC=0;
  state RestFinal
    entry:
    Mode_Cntrl_cap = 3;
    WaitTime =0;
    Step=7;
    during:
    WaitTime = WaitTime + sim_step_time;
  state WaitECUWakeUp
    entry:
    Mode_Cntrl_cap = 3;
    WaitTime = 0;
    Step=8;
    during:
    WaitTime = WaitTime + sim_step_time;
  state Tester
    entry:
    Mode_Cntrl_cap = 3;
    Step=88;
  (default) -> start_test
  Charge -> RestBefore [order 1] : [(Current<=CurrentTerm) && (WaitTime>20)]
  discharge -> Charge [order 1] : [(Current>=(CurrentTerm*-1)) && (WaitTime>20)]
  start_test -> discharge [order 1] : [ (WaitTime>=30)]
  RestBefore -> ResetSOC [order 1] : [WaitTime>=RestTime]
  DischargeIncrement -> RestBetweenResetRun [order 2] : [(Delta >= deltaAhr) && (WaitTime>5)]
  RestBetweenResetRun -> WaitECUWakeUp : [WaitTime>=RestTime]
  DischargeIncrement -> RestFinal [order 1] : [Voltage<= Vfloor]
  ResetSOC -> DischargeIncrement [order 1] : [WaitTime>=20]
  RestFinal -> end_test : [WaitTime>=RestTime]
  WaitECUWakeUp -> DischargeIncrement : [WaitTime>=20]
  start_test -> Tester [order 2] : [Test==1]
  Tester -> discharge [order 2] : [(StepTest==1) && (Test==1)]
  discharge -> Tester [order 2] : [(StepTest~=1 ) && (Test==1)]
  Tester -> Charge [order 3] : [(StepTest == 2) && (Test==1)]
  Charge -> Tester [order 2] : [(StepTest~=2 ) && (Test==1)]
  Tester -> RestBefore [order 4] : [(StepTest==3) && (Test==1)]
  RestBefore -> Tester [order 2] : [(StepTest~=3 ) && (Test==1)]
  Tester -> ResetSOC [order 5] : [(StepTest==4) && (Test==1)]
  ResetSOC -> Tester [order 2] : [(StepTest~=4 ) && (Test==1)]
  Tester -> DischargeIncrement [order 6] : [(StepTest==5) && (Test==1)]
  DischargeIncrement -> Tester [order 3] : [(StepTest~=5 ) && (Test==1)]
  Tester -> start_test [order 1] : [(StepTest==0) && (Test==0)]
  data: Control_Value_cap output double; Vfloor input single; RateDischrg input single; WaitTime output double; RateChrg input single; Mode_Cntrl_cap output single; Vlid input single; CurrentTerm input single; Voltage input single; Current input single; sim_step_time input single; ChrgCurrLim input single; DischrgCurrLim input single; DischrgCurrLim_Tmp output single; ChrgCurrLim_Tmp output single; Step output single; PackSens input boolean; RateOCVDischrg input double; Ahr input double; AhrOld local double; RestTime input double; deltaAhr input double; ResetSOC output boolean; Delta local double; ResetRun output double; Test input double; StepTest input double

== matlab function LionsHeart/FeaturePresentation/Down_to_Business/DriveProfile_ModeControl/ProfileScheduleBreakout/Class Breakout ==
  data: list input double; item1 output double; item2 output double; item3 output double; item4 output double; item5 output double; item6 output double; item7 output double; item8 output double; item9 output double; item10 output double; item11 output double; item12 output double; item13 output double; item14 output double; item15 output double; item16 output double; item17 output double; item18 output double; item19 output double; item20 output double
function [item1, item2, item3, item4, item5, item6, item7, item8, item9, item10, item11, item12, item13, item14, item15, item16, item17, item18, item19, item20]= breakout20(list)

item1 = list(1);
item2 = list(2);
item3 = list(3);
item4 = list(4);
item5 = list(5);
item6 = list(6);
item7 = list(7);
item8 = list(8);
item9 = list(9);
item10 = list(10);
item11 = list(11);
item12 = list(12);
item13 = list(13);
item14 = list(14);
item15 = list(15);
item16 = list(16);
item17 = list(17);
item18 = list(18);
item19 = list(19);
item20 = list(20);

end

== matlab function LionsHeart/FeaturePresentation/Down_to_Business/DriveProfile_ModeControl/ProfileScheduleBreakout/Parameter Breakout ==
  data: list input double; item1 output double; item2 output double; item3 output double; item4 output double; item5 output double; item6 output double; item7 output double; item8 output double; item9 output double; item10 output double; item11 output double; item12 output double; item13 output double; item14 output double; item15 output double; item16 output double; item17 output double; item18 output double; item19 output double; item20 output double
function [item1, item2, item3, item4, item5, item6, item7, item8, item9, item10, item11, item12, item13, item14, item15, item16, item17, item18, item19, item20]= breakout20(list)

item1 = list(1);
item2 = list(2);
item3 = list(3);
item4 = list(4);
item5 = list(5);
item6 = list(6);
item7 = list(7);
item8 = list(8);
item9 = list(9);
item10 = list(10);
item11 = list(11);
item12 = list(12);
item13 = list(13);
item14 = list(14);
item15 = list(15);
item16 = list(16);
item17 = list(17);
item18 = list(18);
item19 = list(19);
item20 = list(20);

end

== matlab function LionsHeart/FeaturePresentation/Down_to_Business/DriveProfile_ModeControl/ProfileScheduleBreakout/Type Breakout ==
  data: list input double; item1 output double; item2 output double; item3 output double; item4 output double; item5 output double; item6 output double; item7 output double; item8 output double; item9 output double; item10 output double; item11 output double; item12 output double; item13 output double; item14 output double; item15 output double; item16 output double; item17 output double; item18 output double; item19 output double; item20 output double
function [item1, item2, item3, item4, item5, item6, item7, item8, item9, item10, item11, item12, item13, item14, item15, item16, item17, item18, item19, item20]= breakout20(list)

item1 = list(1);
item2 = list(2);
item3 = list(3);
item4 = list(4);
item5 = list(5);
item6 = list(6);
item7 = list(7);
item8 = list(8);
item9 = list(9);
item10 = list(10);
item11 = list(11);
item12 = list(12);
item13 = list(13);
item14 = list(14);
item15 = list(15);
item16 = list(16);
item17 = list(17);
item18 = list(18);
item19 = list(19);
item20 = list(20);

end
